simulink model "digital_example"  (R2019b)
settings: Solver=VariableStepAuto  StartTime=0.0  StopTime=2  MaxStep=0.001  RelTol=1e-3
values from neighbouring files (symbols this model uses):
  Kp = 1/(2*Tu*K1*K2)    [P-regul.m]    (also in P_regul.m)
  T0 = 1    [P-regul.m]    (also in P_regul.m)
settings Model: Creator=Anton Mayorov  LastModifiedBy=bedla
settings DataIOCC: ReturnWorkspaceOutputs=off
settings DebuggingCC: ArithmeticOperatorsInVariantConditions=warning
settings SFSimCC: SimUseLocalCustomCode=off  CustomCodeUndefinedFunction=UseInterfaceOnly
settings RTWCC: RTWUseLocalCustomCode=off

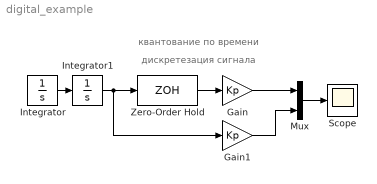
== system digital_example ==
  note: дискретезация сигнала
  note: квантование по времени
  Gain : Gain  Gain=Kp
  Gain1 : Gain  Gain=Kp
  Integrator : Integrator  InitialCondition=1
  Integrator1 : Integrator
  Mux : Mux  Inputs=2
  Scope : Scope
  Zero-Order Hold : ZeroOrderHold  SampleTime=T0
  wires:
  Integrator/1 -> Integrator1/1
  Integrator1/1 -> Gain1/1, Zero-Order Hold/1
  Zero-Order Hold/1 -> Gain/1
  Gain/1 -> Mux/1
  Mux/1 -> Scope/1
  Gain1/1 -> Mux/2
